simulink model "soc"  (R2025b)
settings: Solver=FixedStepDiscrete  StartTime=0.0  StopTime=10  FixedStep=0.01  RelTol=1e-3
PreLoadFcn:
  | % === Get the current model's directory ===
  | modelFullPath = get_param(bdroot, 'FileName');
  | modelDir = fileparts(modelFullPath);
  | 
  | 
  | % === Get the project root folder ===
  | projectRoot = fileparts(modelDir);
  | 
  | 
  | % === Add key folders to path ===
  | addpath(fullfile(projectRoot, 'ReferenceSubsystems'));
  | %addpath(fullfile(projectRoot, 'Docs'));
  | addpath(fullfile(projectRoot, 'design'));
  | 
  | 
  | % Load lookup table script
  | %run('Lookuptable.m');
  | 
  | 
  | 
  | 
PostLoadFcn:
  | float32 = Simulink.AliasType;
  | 
  | float32.BaseType = 'single';
  | 
  | float32.HeaderFile = 'Platform_Types.h';
  | 
  | assignin('base', 'float32', float32);
values from neighbouring files (symbols this model uses):
  Battsm_State_t : value not decoded    [soc.sldd]
  FRACTION_TO_PERCENT = 100.0    [soc.sldd]
  KeSoc_A_RestingCurrent = 4.0    [soc.sldd]
  KeSoc_frc_BotmOfDchRst = 0.0    [soc.sldd]
  KeSoc_frc_LowSocResetThd = 0.12    [soc.sldd]
  KeSoc_frc_LowSocSetThd = 0.1    [soc.sldd]
  KeSoc_frc_SocMaxLim = 1.0    [soc.sldd]
  KeSoc_frc_SocMinLim = 0.0    [soc.sldd]
  KeSoc_frc_TopOfChrgRst = 1.0    [soc.sldd]
  KeSoc_frc_UserSocMaxLim = 0.99    [soc.sldd]
  KeSoc_frc_UserSocMinLim = 0.014    [soc.sldd]
  KeSoc_nu_EpsVal = 2.2204460492503131E-16    [soc.sldd]
  KeSoc_nu_RestTauFactor = 3.0    [soc.sldd]
  KeSoc_sec_SampleTime = 0.01    [soc.sldd]
  KeSoc_sec_SocBodSetTime = 0.0    [soc.sldd]
  KeSoc_sec_SocTocSetTime = 0.0    [soc.sldd]
  KeSoc_V_BodMinCellVolt = 2.993    [soc.sldd]
  KeSoc_V_TocAvrgCellVolt = 4.5    [soc.sldd]
  KeSoc_V_TocMaxCellVolt = 4.5    [soc.sldd]
  PERCENT_TO_FRACTION = 0.01    [soc.sldd]
  SEC_TO_MILLISEC = 1000.0    [soc.sldd]
  SOC_NUM_OF_CELLS = 8.0    [soc.sldd]
  Soc_State_t : value not decoded    [soc.sldd]
libraries: simulink x25
(part 1 of 2)
settings Model: DataDictionary=soc.sldd  Creator=Niharika  LastModifiedBy=Niharika
settings OptimizationCC: BlockReduction=off  DefaultParameterBehavior=Inlined  UseDivisionForNetSlopeComputation=on  DefaultUnderspecifiedDataType=single  EnhancedBackFolding=on  PassReuseOutputArgsAs=Individual arguments  EfficientFloat2IntCast=on  LifeSpan=inf  OptimizeBlockOrder=speed  DifferentSizesBufferReuse=on  OptimizationCustomize=off  EfficientTunableParamExpr=on
settings DebuggingCC: SignalInfNanChecking=error  ReadBeforeWriteMsg=EnableAllAsError  WriteAfterWriteMsg=EnableAllAsError  WriteAfterReadMsg=EnableAllAsError  AlgebraicLoopMsg=error  ArtificialAlgebraicLoopMsg=error  SaveWithDisabledLinksMsg=error  SaveWithParameterizedLinksMsg=error  BlockPriorityViolationMsg=error  SolverPrmCheckMsg=error  SingleTaskRateTransMsg=warning  CheckMatrixSingularityMsg=error  IntegerOverflowMsg=error  ParameterOverflowMsg=none  ParameterPrecisionLossMsg=none  ParameterTunabilityLossMsg=none  UnnecessaryDatatypeConvMsg=warning  SignalLabelMismatchMsg=error  UnconnectedInputMsg=error  UnconnectedOutputMsg=error  UnconnectedLineMsg=error  SFcnCompatibilityMsg=error  UniqueDataStoreMsg=error  BusObjectLabelMismatch=error  RootOutportRequireBusObject=error  AssertControl=DisableAll  ModelReferenceIOMismatchMessage=error  ModelReferenceDataLoggingMessage=error  StateNameClashWarn=warning  StrictBusMsg=ErrorOnBusTreatedAsVector  NonBusSignalsTreatedAsBus=error  SFInvalidInputDataAccessInChartInitDiag=error  SFTransitionOutsideNaturalParentDiag=error  SFUnreachableExecutionPathDiag=error  SFUndirectedBroadcastEventsDiag=error  SFTransitionActionBeforeConditionDiag=error  SFTemporalDelaySmallerThanSampleTimeDiag=error  SFSelfTransitionDiag=error  SFExecutionAtInitializationDiag=error  IntegerSaturationMsg=error  UnderSpecifiedDimensionMsg=warning  VariantConditionMismatch=error
settings HardwareCC: ProdBitPerPointer=32.0  ProdBitPerSizeT=32.0  ProdBitPerPtrDiffT=32.0  ProdLargestAtomicInteger=Long  ProdLargestAtomicFloat=Double  ProdWordSize=32.0  ProdHWDeviceType=ARM Compatible->ARM Cortex-M
settings SFSimCC: SimGenImportedTypeDefs=on  CompileTimeRecursionLimit=0.0  EnableRuntimeRecursion=off  MATLABDynamicMemAlloc=off
settings RTWCC: SystemTargetFile=ert.tlc  GenCodeOnly=on  TemplateMakefile=ert_default_tmf  DataTypeReplacement=CDataTypesFixedWidth  GPUComputeCapability=3.5  Description=Embedded Coder
settings CodeAppCC: ForceParamTrailComments=on  IgnoreCustomStorageClasses=off  IgnoreTestpoints=on  OperatorAnnotations=on  SimulinkDataObjDesc=on  SFDataObjDesc=on  MATLABFcnDesc=on  MangleLength=4.0  CustomUserTokenString=model  InsertBlockDesc=on  ReqsInCode=on
settings ERTTargetCC: MultiInstanceErrorCode=None  ERTCustomFileTemplate=example_file_process.tlc  GlobalDataReference=InSourceFile  ERTFilePackagingFormat=Compact  PreserveExpressionOrder=on  EnableSignedLeftShifts=off  EnableSignedRightShifts=off  IndentStyle=Allman  IndentSize=4  EnableUserReplacementTypes=on  MaxIdInt64=INT64_MAX  MinIdInt64=INT64_MIN  MaxIdUint64=UINT64_MAX  MaxIdInt32=INT32_MAX  MinIdInt32=INT32_MIN  MaxIdUint32=UINT32_MAX  MaxIdInt16=INT16_MAX  MinIdInt16=INT16_MIN  MaxIdUint16=UINT16_MAX  MaxIdInt8=INT8_MAX  MinIdInt8=INT8_MIN  MaxIdUint8=UINT8_MAX  DynamicArrayContainerType=coder::array  TargetLangStandard=C99 (ISO)  GenerateFullHeader=off  IncludeMdlTerminateFcn=off  SuppressErrorStatus=on  ERTCustomFileBanners=off  SupportAbsoluteTime=off  SupportNonFinite=off  SupportComplex=off  ParenthesesLevel=Standards  CastingMode=Standards  GenerateSharedConstants=off  ERTHeaderFileRootName=$R$U$E  ERTSourceFileRootName=$R$U$E
settings ConfigComp: CovScope=ReferencedModels  DVMaxProcessTime=300.0  DVMaxTestCaseSteps=10000.0  DVTestSuiteOptimization=Auto  DVAbsoluteTolerance=1.0e-5  DVDefectChecker=off  DVDetectOutOfBounds=on  DVDesignMinMaxCheck=on  DVDetectDSMAccessViolations=on  DVDetectHISMViolationsHisl_0002=on  DVDetectHISMViolationsHisl_0003=on  DVDetectHISMViolationsHisl_0004=on  DVDetectHISMViolationsHisl_0028=on  DVDetectBlockInputRangeViolations=on  DVMaxViolationSteps=20.0  DVModelReferenceHarness=on  DVHarnessSource=Signal Editor  DVActiveTab=0.0

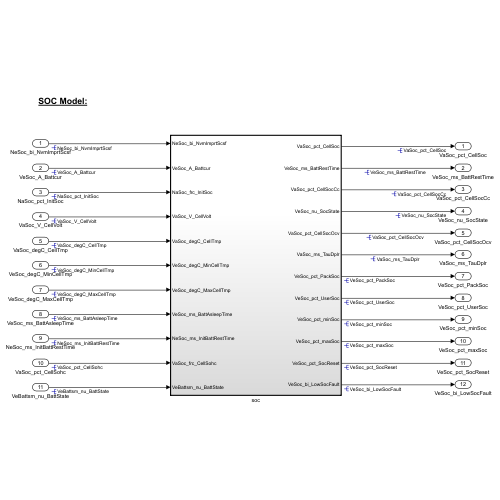
[thumbnail: Simulink's stored preview of the top-level diagram]
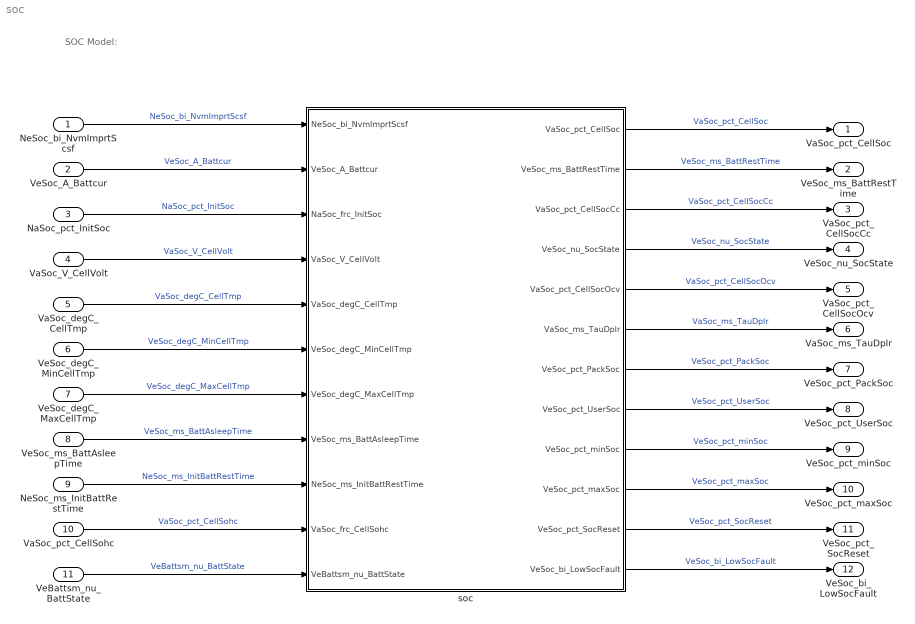
== system soc ==
  note: SOC Model:
  NeSoc_bi_NvmImprtScsf : Inport  OutMin=0  OutMax=1  OutDataTypeStr=boolean  PortDimensions=[1]  SampleTime=0.01
  VeSoc_A_Battcur : Inport  Port=2  OutMin=-6000  OutMax=6000  OutDataTypeStr=single  Unit=mA  PortDimensions=[1]  SampleTime=0.01
  NaSoc_pct_InitSoc : Inport  Port=3  OutDataTypeStr=single  PortDimensions=[1,SOC_NUM_OF_CELLS]  SampleTime=0.01
  VaSoc_V_CellVolt : Inport  Port=4  OutMin=2  OutMax=5  OutDataTypeStr=single  PortDimensions=[1,SOC_NUM_OF_CELLS]  SampleTime=0.01
  VaSoc_degC_CellTmp : Inport  Port=5  OutMin=-35  OutMax=60  OutDataTypeStr=single  Unit=degC  PortDimensions=[1,SOC_NUM_OF_CELLS]  SampleTime=0.01
  VeSoc_degC_MinCellTmp : Inport  Port=6  OutMin=-35  OutMax=60  OutDataTypeStr=single  Unit=degC  PortDimensions=[1]  SampleTime=0.01
  VeSoc_degC_MaxCellTmp : Inport  Port=7  OutMin=-35  OutMax=60  OutDataTypeStr=single  Unit=degC  PortDimensions=[1]  SampleTime=0.01
  VeSoc_ms_BattAsleepTime : Inport  Port=8  OutDataTypeStr=uint32  Unit=ms  PortDimensions=[1]  SampleTime=0.01
  NeSoc_ms_InitBattRestTime : Inport  Port=9  OutDataTypeStr=uint32  Unit=ms  PortDimensions=[1]  SampleTime=0.01
  VaSoc_pct_CellSohc : Inport  Port=10  OutMin=0.01  OutDataTypeStr=single  PortDimensions=[1,SOC_NUM_OF_CELLS]  SampleTime=0.01
  VeBattsm_nu_BattState : Inport  Port=11  OutDataTypeStr=Enum: Battsm_State_t  PortDimensions=[1]  SampleTime=0.01
  soc : Subsystem  Description=SOC Estimation Algorithm Main/Top level subsystem  TreatAsAtomicUnit=on
      settings: RTWSystemCode=Inline
  VaSoc_pct_CellSoc : Outport  OutDataTypeStr=single  PortDimensions=[1,SOC_NUM_OF_CELLS]  SampleTime=0.01
  VeSoc_ms_BattRestTime : Outport  Port=2  OutDataTypeStr=uint32  PortDimensions=[1]  SampleTime=0.01
  VaSoc_pct_CellSocCc : Outport  Port=3  OutDataTypeStr=single  PortDimensions=[1,SOC_NUM_OF_CELLS]  SampleTime=0.01
  VeSoc_nu_SocState : Outport  Port=4  OutDataTypeStr=Enum: Soc_State_t  PortDimensions=[1]  SampleTime=0.01
  VaSoc_pct_CellSocOcv : Outport  Port=5  OutDataTypeStr=single  PortDimensions=[1,SOC_NUM_OF_CELLS]  SampleTime=0.01
  VaSoc_ms_TauDplr : Outport  Port=6  OutDataTypeStr=single  PortDimensions=[1,SOC_NUM_OF_CELLS]  SampleTime=0.01
  VeSoc_pct_PackSoc : Outport  Port=7  OutDataTypeStr=single  SampleTime=0.01
  VeSoc_pct_UserSoc : Outport  Port=8  OutDataTypeStr=single  SampleTime=0.01
  VeSoc_pct_minSoc : Outport  Port=9
  VeSoc_pct_maxSoc : Outport  Port=10
  VeSoc_pct_SocReset : Outport  Port=11
  VeSoc_bi_LowSocFault : Outport  Port=12
  wires:
  soc/2(VeSoc_ms_BattRestTime) -> VeSoc_ms_BattRestTime/1  "VeSoc_ms_BattRestTime"
  soc/6(VaSoc_ms_TauDplr) -> VaSoc_ms_TauDplr/1  "VaSoc_ms_TauDplr"
  soc/3(VaSoc_pct_CellSocCc) -> VaSoc_pct_CellSocCc/1  "VaSoc_pct_CellSocCc"
  soc/5(VaSoc_pct_CellSocOcv) -> VaSoc_pct_CellSocOcv/1  "VaSoc_pct_CellSocOcv"
  soc/1(VaSoc_pct_CellSoc) -> VaSoc_pct_CellSoc/1  "VaSoc_pct_CellSoc"
  soc/4(VeSoc_nu_SocState) -> VeSoc_nu_SocState/1  "VeSoc_nu_SocState"
  soc/7(VeSoc_pct_PackSoc) -> VeSoc_pct_PackSoc/1  "VeSoc_pct_PackSoc"
  soc/8(VeSoc_pct_UserSoc) -> VeSoc_pct_UserSoc/1  "VeSoc_pct_UserSoc"
  soc/10(VeSoc_pct_maxSoc) -> VeSoc_pct_maxSoc/1  "VeSoc_pct_maxSoc"
  soc/11(VeSoc_pct_SocReset) -> VeSoc_pct_SocReset/1  "VeSoc_pct_SocReset"
  soc/12(VeSoc_bi_LowSocFault) -> VeSoc_bi_LowSocFault/1  "VeSoc_bi_LowSocFault"
  soc/9(VeSoc_pct_minSoc) -> VeSoc_pct_minSoc/1  "VeSoc_pct_minSoc"
  NeSoc_bi_NvmImprtScsf/1 -> soc/1(NeSoc_bi_NvmImprtScsf)  "NeSoc_bi_NvmImprtScsf"
  VeSoc_A_Battcur/1 -> soc/2(VeSoc_A_Battcur)  "VeSoc_A_Battcur"
  NaSoc_pct_InitSoc/1 -> soc/3(NaSoc_frc_InitSoc)  "NaSoc_pct_InitSoc"
  VaSoc_V_CellVolt/1 -> soc/4(VaSoc_V_CellVolt)  "VaSoc_V_CellVolt"
  VaSoc_degC_CellTmp/1 -> soc/5(VaSoc_degC_CellTmp)  "VaSoc_degC_CellTmp"
  VeSoc_degC_MinCellTmp/1 -> soc/6(VeSoc_degC_MinCellTmp)  "VeSoc_degC_MinCellTmp"
  VeSoc_degC_MaxCellTmp/1 -> soc/7(VeSoc_degC_MaxCellTmp)  "VeSoc_degC_MaxCellTmp"
  VeSoc_ms_BattAsleepTime/1 -> soc/8(VeSoc_ms_BattAsleepTime)  "VeSoc_ms_BattAsleepTime"
  NeSoc_ms_InitBattRestTime/1 -> soc/9(NeSoc_ms_InitBattRestTime)  "NeSoc_ms_InitBattRestTime"
  VaSoc_pct_CellSohc/1 -> soc/10(VaSoc_frc_CellSohc)  "VaSoc_pct_CellSohc"
  VeBattsm_nu_BattState/1 -> soc/11(VeBattsm_nu_BattState)  "VeBattsm_nu_BattState"

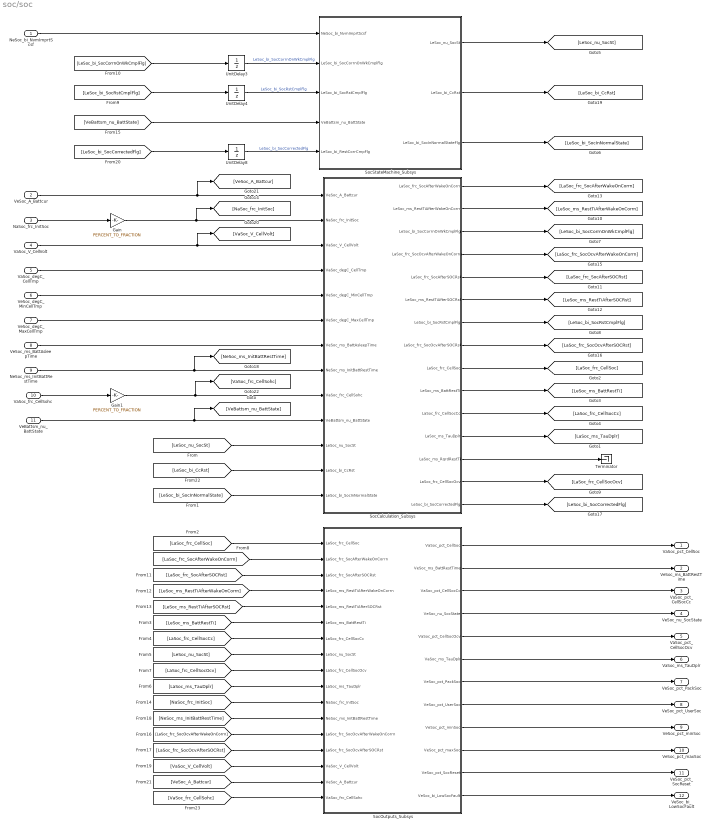
== system soc/soc ==
  NeSoc_bi_NvmImprtScsf : Inport
  VeSoc_A_Battcur : Inport  Port=2
  NaSoc_frc_InitSoc : Inport  Port=3
  VaSoc_V_CellVolt : Inport  Port=4
  VaSoc_degC_CellTmp : Inport  Port=5
  VeSoc_degC_MinCellTmp : Inport  Port=6
  VeSoc_degC_MaxCellTmp : Inport  Port=7
  VeSoc_ms_BattAsleepTime : Inport  Port=8
  NeSoc_ms_InitBattRestTime : Inport  Port=9
  VaSoc_frc_CellSohc : Inport  Port=10
  VeBattsm_nu_BattState : Inport  Port=11
  Gain : Gain  Gain=PERCENT_TO_FRACTION
  Gain1 : Gain  Gain=PERCENT_TO_FRACTION
  SocCalculation_Subsys : Subsystem  TreatAsAtomicUnit=on
  SocOutputs_Subsys : Subsystem  TreatAsAtomicUnit=on
  SocStateMachine_Subsys : Subsystem  TreatAsAtomicUnit=on
  Terminator : Terminator
  UnitDelay3 : UnitDelay  SampleTime=-1  HasFrameUpgradeWarning=on
  UnitDelay4 : UnitDelay  SampleTime=-1  HasFrameUpgradeWarning=on
  UnitDelay8 : UnitDelay  SampleTime=-1  HasFrameUpgradeWarning=on
  VaSoc_pct_CellSoc : Outport
  VeSoc_ms_BattRestTime : Outport  Port=2
  VaSoc_pct_CellSocCc : Outport  Port=3
  VeSoc_nu_SocState : Outport  Port=4
  VaSoc_pct_CellSocOcv : Outport  Port=5
  VaSoc_ms_TauDplr : Outport  Port=6
  VeSoc_pct_PackSoc : Outport  Port=7
  VeSoc_pct_UserSoc : Outport  Port=8
  VeSoc_pct_minSoc : Outport  Port=9
  VeSoc_pct_maxSoc : Outport  Port=10
  VeSoc_pct_SocReset : Outport  Port=11
  VeSoc_bi_LowSocFault : Outport  Port=12
  wires:
  NeSoc_bi_NvmImprtScsf/1 -> SocStateMachine_Subsys/1(NeSoc_bi_NvmImprtScsf)
  NaSoc_frc_InitSoc/1 -> Gain/1
  VaSoc_degC_CellTmp/1 -> SocCalculation_Subsys/4(VaSoc_degC_CellTmp)
  VeSoc_degC_MinCellTmp/1 -> SocCalculation_Subsys/5(VeSoc_degC_MinCellTmp)
  VeSoc_degC_MaxCellTmp/1 -> SocCalculation_Subsys/6(VeSoc_degC_MaxCellTmp)
  VeSoc_ms_BattAsleepTime/1 -> SocCalculation_Subsys/7(VeSoc_ms_BattAsleepTime)
  NeSoc_ms_InitBattRestTime/1 -> [NeSoc_ms_InitBattRestTime], SocCalculation_Subsys/8(NeSoc_ms_InitBattRestTime)
  VaSoc_frc_CellSohc/1 -> Gain1/1
  SocCalculation_Subsys/13(LaSoc_ms_RqrdRestTi) -> Terminator/1
  SocCalculation_Subsys/12(LaSoc_ms_TauDplr) -> [LaSoc_ms_TauDplr]
  SocCalculation_Subsys/6(LeSoc_ms_RestTiAfterSOCRst) -> [LeSoc_ms_RestTiAfterSOCRst]
  SocCalculation_Subsys/11(LaSoc_frc_CellSocCc) -> [LaSoc_frc_CellSocCc]
  SocCalculation_Subsys/10(LeSoc_ms_BattRestTi) -> [LeSoc_ms_BattRestTi]
  SocCalculation_Subsys/2(LeSoc_ms_RestTiAfterWakeOnCorrn) -> [LeSoc_ms_RestTiAfterWakeOnCorrn]
  SocCalculation_Subsys/9(LaSoc_frc_CellSoc) -> [LaSoc_frc_CellSoc]
  SocCalculation_Subsys/14(LaSoc_frc_CellSocOcv) -> [LaSoc_frc_CellSocOcv]
  SocCalculation_Subsys/7(LeSoc_bi_SocRstCmplFlg) -> [LeSoc_bi_SocRstCmplFlg]
  SocCalculation_Subsys/3(LeSoc_bi_SocCorrnOnWkCmplFlg) -> [LeSoc_bi_SocCorrnOnWkCmplFlg]
  SocStateMachine_Subsys/1(LeSoc_nu_SocSt) -> [LeSoc_nu_SocSt]
  VeSoc_A_Battcur/1 -> [VeSoc_A_Battcur], SocCalculation_Subsys/1(VeSoc_A_Battcur)
  VaSoc_V_CellVolt/1 -> [VaSoc_V_CellVolt], SocCalculation_Subsys/3(VaSoc_V_CellVolt)
  [LeSoc_ms_BattRestTi] -> SocOutputs_Subsys/6(LeSoc_ms_BattRestTi)
  SocOutputs_Subsys/5(VaSoc_pct_CellSocOcv) -> VaSoc_pct_CellSocOcv/1
  [LeSoc_ms_RestTiAfterSOCRst] -> SocOutputs_Subsys/5(LeSoc_ms_RestTiAfterSOCRst)
  [LaSoc_frc_SocAfterSOCRst] -> SocOutputs_Subsys/3(LaSoc_frc_SocAfterSOCRst)
  SocOutputs_Subsys/4(VeSoc_nu_SocState) -> VeSoc_nu_SocState/1
  [LaSoc_frc_SocAfterWakeOnCorrn] -> SocOutputs_Subsys/2(LaSoc_frc_SocAfterWakeOnCorrn)
  [LaSoc_frc_CellSocOcv] -> SocOutputs_Subsys/9(LaSoc_frc_CellSocOcv)
  [LeSoc_ms_RestTiAfterWakeOnCorrn] -> SocOutputs_Subsys/4(LeSoc_ms_RestTiAfterWakeOnCorrn)
  [LeSoc_nu_SocSt] -> SocOutputs_Subsys/8(LeSoc_nu_SocSt)
  SocOutputs_Subsys/6(VaSoc_ms_TauDplr) -> VaSoc_ms_TauDplr/1
  [LaSoc_frc_CellSoc] -> SocOutputs_Subsys/1(LaSoc_frc_CellSoc)
  SocOutputs_Subsys/3(VaSoc_pct_CellSocCc) -> VaSoc_pct_CellSocCc/1
  [LaSoc_frc_CellSocCc] -> SocOutputs_Subsys/7(LaSoc_frc_CellSocCc)
  [LaSoc_ms_TauDplr] -> SocOutputs_Subsys/10(LaSoc_ms_TauDplr)
  [LeSoc_bi_SocRstCmplFlg] -> UnitDelay4/1
  [LeSoc_bi_SocCorrnOnWkCmplFlg] -> UnitDelay3/1
  SocCalculation_Subsys/1(LaSoc_frc_SocAfterWakeOnCorrn) -> [LaSoc_frc_SocAfterWakeOnCorrn]
  SocCalculation_Subsys/5(LaSoc_frc_SocAfterSOCRst) -> [LaSoc_frc_SocAfterSOCRst]
  SocOutputs_Subsys/1(VaSoc_pct_CellSoc) -> VaSoc_pct_CellSoc/1
  SocOutputs_Subsys/2(VeSoc_ms_BattRestTime) -> VeSoc_ms_BattRestTime/1
  [VeBattsm_nu_BattState] -> SocStateMachine_Subsys/4(VeBattsm_nu_BattState)
  VeBattsm_nu_BattState/1 -> [VeBattsm_nu_BattState], SocCalculation_Subsys/10(VeBattsm_nu_BattState)
  SocCalculation_Subsys/4(LaSoc_frc_SocOcvAfterWakeOnCorrn) -> [LaSoc_frc_SocOcvAfterWakeOnCorrn]
  SocCalculation_Subsys/8(LaSoc_frc_SocOcvAfterSOCRst) -> [LaSoc_frc_SocOcvAfterSOCRst]
  [LaSoc_frc_SocOcvAfterSOCRst] -> SocOutputs_Subsys/14(LaSoc_frc_SocOcvAfterSOCRst)
  [LaSoc_frc_SocOcvAfterWakeOnCorrn] -> SocOutputs_Subsys/13(LaSoc_frc_SocOcvAfterWakeOnCorrn)
  [LeSoc_nu_SocSt] -> SocCalculation_Subsys/11(LeSoc_nu_SocSt)
  SocCalculation_Subsys/15(LeSoc_bi_SocCorrectedFlg) -> [LeSoc_bi_SocCorrectedFlg]
  [LeSoc_bi_SocCorrectedFlg] -> UnitDelay8/1
  SocStateMachine_Subsys/2(LeSoc_bi_CcRst) -> [LeSoc_bi_CcRst]
  [LeSoc_bi_CcRst] -> SocCalculation_Subsys/12(LeSoc_bi_CcRst)
  UnitDelay3/1 -> SocStateMachine_Subsys/2(LeSoc_bi_SocCorrnOnWkCmplFlg)  "LeSoc_bi_SocCorrnOnWkCmplFlg"
  UnitDelay4/1 -> SocStateMachine_Subsys/3(LeSoc_bi_SocRstCmplFlg)  "LeSoc_bi_SocRstCmplFlg"
  UnitDelay8/1 -> SocStateMachine_Subsys/5(LeSoc_bi_RestCorrCmpFlg)  "LeSoc_bi_SocCorrectedFlg"
  SocStateMachine_Subsys/3(LeSoc_bi_SocInNormalStateFlg) -> [LeSoc_bi_SocInNormalState]
  [LeSoc_bi_SocInNormalState] -> SocCalculation_Subsys/13(LeSoc_bi_SocInNormalState)
  [NaSoc_frc_InitSoc] -> SocOutputs_Subsys/11(NaSoc_frc_InitSoc)
  [NeSoc_ms_InitBattRestTime] -> SocOutputs_Subsys/12(NeSoc_ms_InitBattRestTime)
  [VaSoc_V_CellVolt] -> SocOutputs_Subsys/15(VaSoc_V_CellVolt)
  [VeSoc_A_Battcur] -> SocOutputs_Subsys/16(VeSoc_A_Battcur)
  [VaSoc_frc_CellSohc] -> SocOutputs_Subsys/17(VaSoc_frc_CellSohc)
  SocOutputs_Subsys/7(VeSoc_pct_PackSoc) -> VeSoc_pct_PackSoc/1
  SocOutputs_Subsys/8(VeSoc_pct_UserSoc) -> VeSoc_pct_UserSoc/1
  SocOutputs_Subsys/9(VeSoc_pct_minSoc) -> VeSoc_pct_minSoc/1
  SocOutputs_Subsys/10(VeSoc_pct_maxSoc) -> VeSoc_pct_maxSoc/1
  SocOutputs_Subsys/11(VeSoc_pct_SocReset) -> VeSoc_pct_SocReset/1
  SocOutputs_Subsys/12(VeSoc_bi_LowSocFault) -> VeSoc_bi_LowSocFault/1
  Gain/1 -> [NaSoc_frc_InitSoc], SocCalculation_Subsys/2(NaSoc_frc_InitSoc)
  Gain1/1 -> [VaSoc_frc_CellSohc], SocCalculation_Subsys/9(VaSoc_frc_CellSohc)

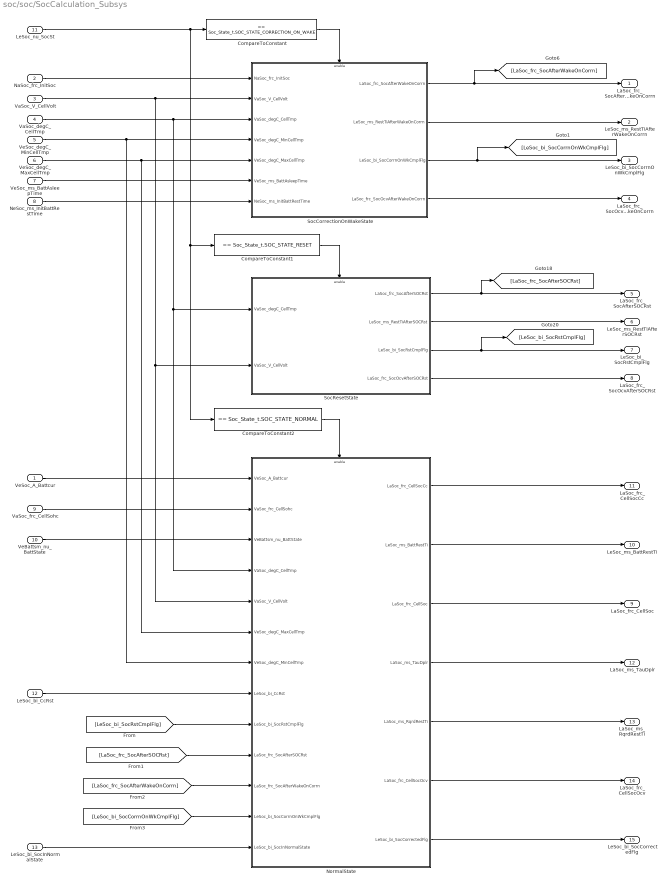
== system soc/soc/SocCalculation_Subsys ==
  VeSoc_A_Battcur : Inport
  NaSoc_frc_InitSoc : Inport  Port=2
  VaSoc_V_CellVolt : Inport  Port=3
  VaSoc_degC_CellTmp : Inport  Port=4
  VeSoc_degC_MinCellTmp : Inport  Port=5
  VeSoc_degC_MaxCellTmp : Inport  Port=6
  VeSoc_ms_BattAsleepTime : Inport  Port=7
  NeSoc_ms_InitBattRestTime : Inport  Port=8
  VaSoc_frc_CellSohc : Inport  Port=9
  VeBattsm_nu_BattState : Inport  Port=10
  LeSoc_nu_SocSt : Inport  Port=11
  LeSoc_bi_CcRst : Inport  Port=12
  LeSoc_bi_SocInNormalState : Inport  Port=13
  CompareToConstant : simulink/Logic and Bit Operations/Compare To Constant  relop===  const=Soc_State_t.SOC_STATE_CORRECTION_ON_WAKE  OutDataTypeStr=boolean
  CompareToConstant1 : simulink/Logic and Bit Operations/Compare To Constant  relop===  const=Soc_State_t.SOC_STATE_RESET  OutDataTypeStr=boolean
  CompareToConstant2 : simulink/Logic and Bit Operations/Compare To Constant  relop===  const=Soc_State_t.SOC_STATE_NORMAL  OutDataTypeStr=boolean
  NormalState : Subsystem  TreatAsAtomicUnit=on
  SocCorrectionOnWakeState : Subsystem  TreatAsAtomicUnit=on
  SocResetState : Subsystem  TreatAsAtomicUnit=on
  LaSoc_frc_SocAfterWakeOnCorrn : Outport
  LeSoc_ms_RestTiAfterWakeOnCorrn : Outport  Port=2
  LeSoc_bi_SocCorrnOnWkCmplFlg : Outport  Port=3
  LaSoc_frc_SocOcvAfterWakeOnCorrn : Outport  Port=4
  LaSoc_frc_SocAfterSOCRst : Outport  Port=5
  LeSoc_ms_RestTiAfterSOCRst : Outport  Port=6
  LeSoc_bi_SocRstCmplFlg : Outport  Port=7
  LaSoc_frc_SocOcvAfterSOCRst : Outport  Port=8
  LaSoc_frc_CellSoc : Outport  Port=9
  LeSoc_ms_BattRestTi : Outport  Port=10
  LaSoc_frc_CellSocCc : Outport  Port=11
  LaSoc_ms_TauDplr : Outport  Port=12
  LaSoc_ms_RqrdRestTi : Outport  Port=13
  LaSoc_frc_CellSocOcv : Outport  Port=14
  LeSoc_bi_SocCorrectedFlg : Outport  Port=15
  wires:
  NaSoc_frc_InitSoc/1 -> SocCorrectionOnWakeState/1(NaSoc_frc_InitSoc)
  VaSoc_V_CellVolt/1 -> SocCorrectionOnWakeState/2(VaSoc_V_CellVolt), SocResetState/2(VaSoc_V_CellVolt), NormalState/5(VaSoc_V_CellVolt)
  VaSoc_degC_CellTmp/1 -> SocCorrectionOnWakeState/3(VaSoc_degC_CellTmp), SocResetState/1(VaSoc_degC_CellTmp), NormalState/4(VaSoc_degC_CellTmp)
  VeSoc_degC_MinCellTmp/1 -> SocCorrectionOnWakeState/4(VeSoc_degC_MinCellTmp), NormalState/7(VeSoc_degC_MinCellTmp)
  VeSoc_degC_MaxCellTmp/1 -> SocCorrectionOnWakeState/5(VeSoc_degC_MaxCellTmp), NormalState/6(VeSoc_degC_MaxCellTmp)
  VeSoc_ms_BattAsleepTime/1 -> SocCorrectionOnWakeState/6(VeSoc_ms_BattAsleepTime)
  NeSoc_ms_InitBattRestTime/1 -> SocCorrectionOnWakeState/7(NeSoc_ms_InitBattRestTime)
  VeSoc_A_Battcur/1 -> NormalState/1(VeSoc_A_Battcur)
  VaSoc_frc_CellSohc/1 -> NormalState/2(VaSoc_frc_CellSohc)
  VeBattsm_nu_BattState/1 -> NormalState/3(VeBattsm_nu_BattState)
  LeSoc_nu_SocSt/1 -> CompareToConstant2/1, CompareToConstant1/1, CompareToConstant/1
  CompareToConstant/1 -> SocCorrectionOnWakeState/Enable
  CompareToConstant1/1 -> SocResetState/Enable
  CompareToConstant2/1 -> NormalState/Enable
  NormalState/6(LaSoc_frc_CellSocOcv) -> LaSoc_frc_CellSocOcv/1
  SocCorrectionOnWakeState/3(LeSoc_bi_SocCorrnOnWkCmplFlg) -> LeSoc_bi_SocCorrnOnWkCmplFlg/1, [LeSoc_bi_SocCorrnOnWkCmplFlg]
  SocResetState/3(LeSoc_bi_SocRstCmplFlg) -> LeSoc_bi_SocRstCmplFlg/1, [LeSoc_bi_SocRstCmplFlg]
  NormalState/5(LaSoc_ms_RqrdRestTi) -> LaSoc_ms_RqrdRestTi/1
  NormalState/1(LaSoc_frc_CellSocCc) -> LaSoc_frc_CellSocCc/1
  NormalState/2(LeSoc_ms_BattRestTi) -> LeSoc_ms_BattRestTi/1
  NormalState/3(LaSoc_frc_CellSoc) -> LaSoc_frc_CellSoc/1
  SocCorrectionOnWakeState/2(LeSoc_ms_RestTiAfterWakeOnCorrn) -> LeSoc_ms_RestTiAfterWakeOnCorrn/1
  SocCorrectionOnWakeState/1(LaSoc_frc_SocAfterWakeOnCorrn) -> LaSoc_frc_SocAfterWakeOnCorrn/1, [LaSoc_frc_SocAfterWakeOnCorrn]
  SocResetState/1(LaSoc_frc_SocAfterSOCRst) -> LaSoc_frc_SocAfterSOCRst/1, [LaSoc_frc_SocAfterSOCRst]
  NormalState/4(LaSoc_ms_TauDplr) -> LaSoc_ms_TauDplr/1
  SocResetState/2(LeSoc_ms_RestTiAfterSOCRst) -> LeSoc_ms_RestTiAfterSOCRst/1
  SocCorrectionOnWakeState/4(LaSoc_frc_SocOcvAfterWakeOnCorrn) -> LaSoc_frc_SocOcvAfterWakeOnCorrn/1
  SocResetState/4(LaSoc_frc_SocOcvAfterSOCRst) -> LaSoc_frc_SocOcvAfterSOCRst/1
  NormalState/7(LeSoc_bi_SocCorrectedFlg) -> LeSoc_bi_SocCorrectedFlg/1
  LeSoc_bi_CcRst/1 -> NormalState/8(LeSoc_bi_CcRst)
  [LeSoc_bi_SocRstCmplFlg] -> NormalState/9(LeSoc_bi_SocRstCmplFlg)
  [LaSoc_frc_SocAfterSOCRst] -> NormalState/10(LaSoc_frc_SocAfterSOCRst)
  [LaSoc_frc_SocAfterWakeOnCorrn] -> NormalState/11(LaSoc_frc_SocAfterWakeOnCorrn)
  [LeSoc_bi_SocCorrnOnWkCmplFlg] -> NormalState/12(LeSoc_bi_SocCorrnOnWkCmplFlg)
  LeSoc_bi_SocInNormalState/1 -> NormalState/13(LeSoc_bi_SocInNormalState)

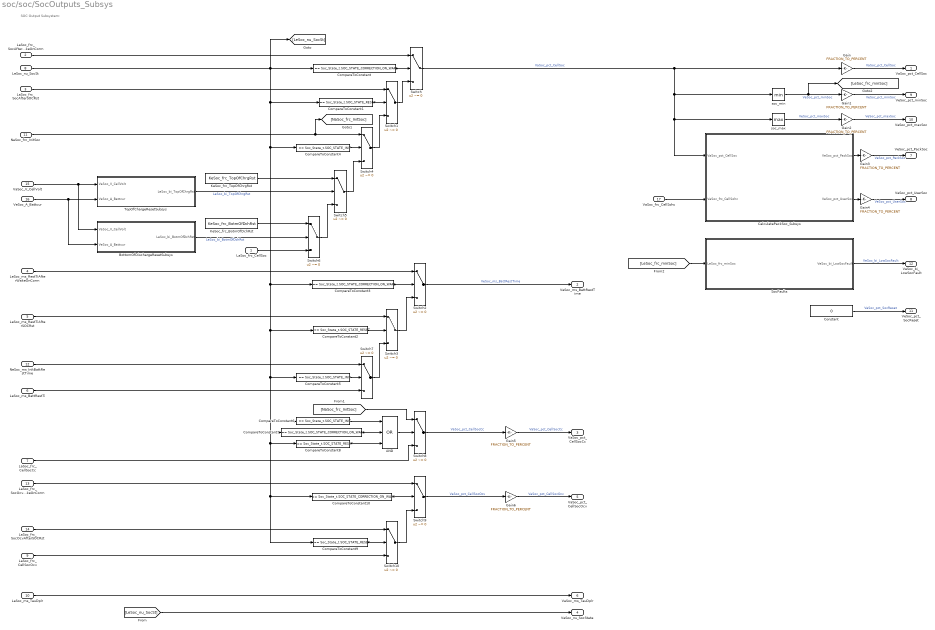
== system soc/soc/SocOutputs_Subsys ==
  note: SOC Output Subsystem:
  LaSoc_frc_CellSoc : Inport
  LaSoc_frc_SocAfterWakeOnCorrn : Inport  Port=2
  LaSoc_frc_SocAfterSOCRst : Inport  Port=3
  LeSoc_ms_RestTiAfterWakeOnCorrn : Inport  Port=4
  LeSoc_ms_RestTiAfterSOCRst : Inport  Port=5
  LeSoc_ms_BattRestTi : Inport  Port=6
  LaSoc_frc_CellSocCc : Inport  Port=7
  LeSoc_nu_SocSt : Inport  Port=8
  LaSoc_frc_CellSocOcv : Inport  Port=9
  LaSoc_ms_TauDplr : Inport  Port=10
  NaSoc_frc_InitSoc : Inport  Port=11
  NeSoc_ms_InitBattRestTime : Inport  Port=12
  LaSoc_frc_SocOcvAfterWakeOnCorrn : Inport  Port=13
  LaSoc_frc_SocOcvAfterSOCRst : Inport  Port=14
  VaSoc_V_CellVolt : Inport  Port=15
  VeSoc_A_Battcur : Inport  Port=16
  VaSoc_frc_CellSohc : Inport  Port=17
  AND : Logic  Operator=OR  Inputs=3  AllPortsSameDT=off  OutDataTypeStr=boolean
  BottomOfDischargeResetSubsys : Subsystem
  CalculatePackSoc_Subsys : Subsystem
  CompareToConstant{,3,7,10} (4 alike) : simulink/Logic and Bit Operations/Compare To Constant  relop===  const=Soc_State_t.SOC_STATE_CORRECTION_ON_WAKE  OutDataTypeStr=boolean
  CompareToConstant{1..2,8..9} (4 alike) : simulink/Logic and Bit Operations/Compare To Constant  relop===  const=Soc_State_t.SOC_STATE_RESET  OutDataTypeStr=boolean
  CompareToConstant4 : simulink/Logic and Bit Operations/Compare To Constant  relop===  const=Soc_State_t.SOC_STATE_INIT  OutDataTypeStr=boolean
  CompareToConstant5 : simulink/Logic and Bit Operations/Compare To Constant  relop===  const=Soc_State_t.SOC_STATE_INIT  OutDataTypeStr=boolean
  CompareToConstant6 : simulink/Logic and Bit Operations/Compare To Constant  relop===  const=Soc_State_t.SOC_STATE_INIT  OutDataTypeStr=boolean
  Constant : Constant  Value=0  OutDataTypeStr=single
  Gain{,1..4} (5 alike) : Gain  Gain=FRACTION_TO_PERCENT  OutDataTypeStr=single
  Gain5 : Gain  Gain=FRACTION_TO_PERCENT
  Gain6 : Gain  Gain=FRACTION_TO_PERCENT
  KeSoc_frc_BotmOfDchRst : Constant  Value=KeSoc_frc_BotmOfDchRst
  KeSoc_frc_TopOfChrgRst : Constant  Value=KeSoc_frc_TopOfChrgRst
  SocFaults : Subsystem
  Switch{,1..10} (11 alike) : Switch  Criteria=u2 ~= 0  SaturateOnIntegerOverflow=off  InputSameDT=off
  TopOfChargeResetSubsys : Subsystem
  soc_max : MinMax  Function=max
  soc_min : MinMax
  VaSoc_pct_CellSoc : Outport
  VeSoc_ms_BattRestTime : Outport  Port=2
  VaSoc_pct_CellSocCc : Outport  Port=3
  VeSoc_nu_SocState : Outport  Port=4
  VaSoc_pct_CellSocOcv : Outport  Port=5
  VaSoc_ms_TauDplr : Outport  Port=6
  VeSoc_pct_PackSoc : Outport  Port=7
  VeSoc_pct_UserSoc : Outport  Port=8
  VeSoc_pct_minSoc : Outport  Port=9
  VeSoc_pct_maxSoc : Outport  Port=10
  VeSoc_pct_SocReset : Outport  Port=11
  VeSoc_bi_LowSocFault : Outport  Port=12
  wires:
  LaSoc_ms_TauDplr/1 -> VaSoc_ms_TauDplr/1
  CompareToConstant/1 -> Switch/2
  LaSoc_frc_SocAfterWakeOnCorrn/1 -> Switch/1
  Switch1/1 -> Switch/3
  CompareToConstant1/1 -> Switch1/2
  LaSoc_frc_SocAfterSOCRst/1 -> Switch1/1
  Switch/1 -> CalculatePackSoc_Subsys/1(VaSoc_pct_CellSoc), soc_max/1, soc_min/1, Gain/1  "VaSoc_pct_CellSoc"
  CompareToConstant2/1 -> Switch3/2
  CompareToConstant3/1 -> Switch2/2
  LeSoc_ms_RestTiAfterWakeOnCorrn/1 -> Switch2/1
  LeSoc_nu_SocSt/1 -> CompareToConstant/1, CompareToConstant3/1, CompareToConstant9/1, CompareToConstant10/1, CompareToConstant8/1, CompareToConstant7/1, CompareToConstant6/1, CompareToConstant5/1, CompareToConstant2/1, CompareToConstant4/1, CompareToConstant1/1, [LeSoc_nu_SocSt]
  LeSoc_ms_RestTiAfterSOCRst/1 -> Switch3/1
  Switch4/1 -> Switch1/3
  [LeSoc_nu_SocSt] -> VeSoc_nu_SocState/1
  Switch2/1 -> VeSoc_ms_BattRestTime/1  "VeSoc_ms_BattRestTime"
  Switch3/1 -> Switch2/3
  Switch7/1 -> Switch3/3
  CompareToConstant5/1 -> Switch7/2
  NaSoc_frc_InitSoc/1 -> [NaSoc_frc_InitSoc], Switch4/1
  CompareToConstant4/1 -> Switch4/2
  LeSoc_ms_BattRestTi/1 -> Switch7/3
  NeSoc_ms_InitBattRestTime/1 -> Switch7/1
  Switch8/1 -> Gain5/1  "VaSoc_pct_CellSocCc"
  AND/1 -> Switch8/2
  CompareToConstant6/1 -> AND/1
  CompareToConstant7/1 -> AND/2
  [NaSoc_frc_InitSoc] -> Switch8/1
  LaSoc_frc_CellSocCc/1 -> Switch8/3
  CompareToConstant8/1 -> AND/3
  CompareToConstant9/1 -> Switch10/2
  LaSoc_frc_CellSocOcv/1 -> Switch10/3
  LaSoc_frc_SocOcvAfterWakeOnCorrn/1 -> Switch9/1
  Switch9/1 -> Gain6/1  "VaSoc_pct_CellSocOcv"
  CompareToConstant10/1 -> Switch9/2
  LaSoc_frc_SocOcvAfterSOCRst/1 -> Switch10/1
  Switch10/1 -> Switch9/3
  Switch5/1 -> Switch4/3
  KeSoc_frc_TopOfChrgRst/1 -> Switch5/1
  TopOfChargeResetSubsys/1(LeSoc_bi_TopOfChrgRst) -> Switch5/2  "LeSoc_bi_TopOfChrgRst"
  Switch6/1 -> Switch5/3
  KeSoc_frc_BotmOfDchRst/1 -> Switch6/1
  BottomOfDischargeResetSubsys/1(LeSoc_bi_BotmOfDchRst) -> Switch6/2  "LeSoc_bi_BotmOfDchRst"
  VaSoc_V_CellVolt/1 -> BottomOfDischargeResetSubsys/1(VaSoc_V_CellVolt), TopOfChargeResetSubsys/1(VaSoc_V_CellVolt)
  VeSoc_A_Battcur/1 -> BottomOfDischargeResetSubsys/2(VeSoc_A_Battcur), TopOfChargeResetSubsys/2(VeSoc_A_Battcur)
  LaSoc_frc_CellSoc/1 -> Switch6/3
  VaSoc_frc_CellSohc/1 -> CalculatePackSoc_Subsys/2(VaSoc_frc_CellSohc)
  CalculatePackSoc_Subsys/1(VeSoc_pct_PackSoc) -> Gain3/1
  CalculatePackSoc_Subsys/2(VeSoc_pct_UserSoc) -> Gain4/1
  soc_min/1 -> [LeSoc_frc_minSoc], Gain1/1  "VeSoc_pct_minSoc"
  soc_max/1 -> Gain2/1  "VeSoc_pct_maxSoc"
  Constant/1 -> VeSoc_pct_SocReset/1  "VeSoc_pct_SocReset"
  Gain/1 -> VaSoc_pct_CellSoc/1  "VaSoc_pct_CellSoc"
  Gain1/1 -> VeSoc_pct_minSoc/1  "VeSoc_pct_minSoc"
  Gain2/1 -> VeSoc_pct_maxSoc/1  "VeSoc_pct_maxSoc"
  Gain3/1 -> VeSoc_pct_PackSoc/1  "VeSoc_pct_PackSoc"
  Gain4/1 -> VeSoc_pct_UserSoc/1  "VeSoc_pct_UserSoc"
  Gain5/1 -> VaSoc_pct_CellSocCc/1  "VaSoc_pct_CellSocCc"
  Gain6/1 -> VaSoc_pct_CellSocOcv/1  "VaSoc_pct_CellSocOcv"
  SocFaults/1(VeSoc_bi_LowSocFault) -> VeSoc_bi_LowSocFault/1  "VeSoc_bi_LowSocFault"
  [LeSoc_frc_minSoc] -> SocFaults/1(LeSoc_frc_minSoc)

== system soc/soc/SocStateMachine_Subsys ==
  note: SOC State Machine Top Level:
  NeSoc_bi_NvmImprtScsf : Inport
  LeSoc_bi_SocCorrnOnWkCmplFlg : Inport  Port=2
  LeSoc_bi_SocRstCmplFlg : Inport  Port=3
  VeBattsm_nu_BattState : Inport  Port=4
  LeSoc_bi_RestCorrCmpFlg : Inport  Port=5
  SOC_StateMachine_Chart : Stateflow chart  TreatAsAtomicUnit=on
  LeSoc_nu_SocSt : Outport
  LeSoc_bi_CcRst : Outport  Port=2  OutDataTypeStr=boolean
  LeSoc_bi_SocInNormalStateFlg : Outport  Port=3
  wires:
  LeSoc_bi_SocRstCmplFlg/1 -> SOC_StateMachine_Chart/3(LeSoc_bi_SocRstCmplFlg)
  SOC_StateMachine_Chart/1(LeSoc_nu_SocSt) -> LeSoc_nu_SocSt/1
  LeSoc_bi_SocCorrnOnWkCmplFlg/1 -> SOC_StateMachine_Chart/2(LeSoc_bi_SocCorrnOnWkCmplFlg)
  NeSoc_bi_NvmImprtScsf/1 -> SOC_StateMachine_Chart/1(NeSoc_bi_NvmImprtScsf)
  VeBattsm_nu_BattState/1 -> SOC_StateMachine_Chart/4(VeBattsm_nu_BattState)
  LeSoc_bi_RestCorrCmpFlg/1 -> SOC_StateMachine_Chart/5(LeSoc_bi_RestCorrCmpFlg)
  SOC_StateMachine_Chart/2(LeSoc_bi_CcRst) -> LeSoc_bi_CcRst/1
  SOC_StateMachine_Chart/3(LeSoc_bi_SocInNormalStateFlg) -> LeSoc_bi_SocInNormalStateFlg/1

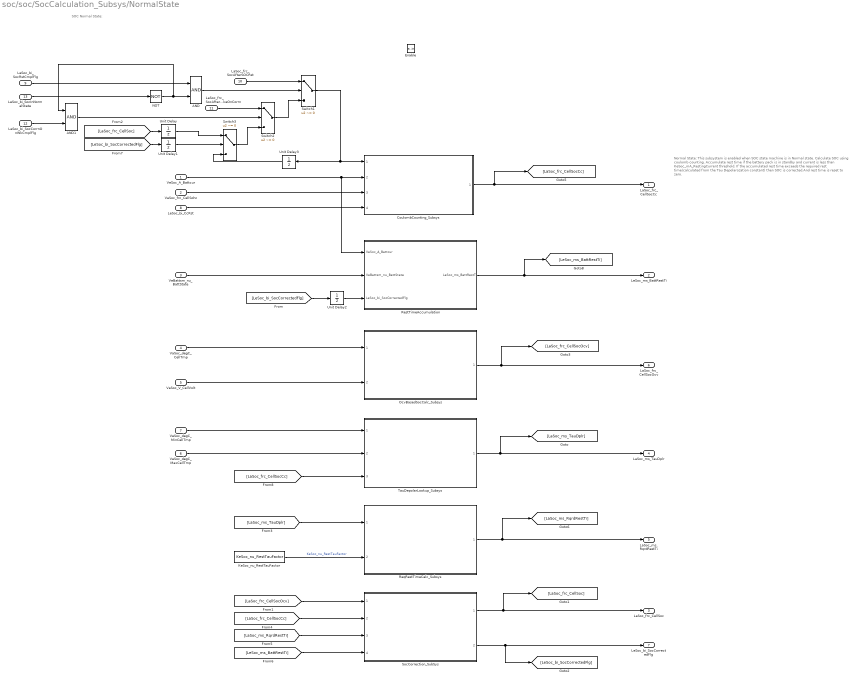
== system soc/soc/SocCalculation_Subsys/NormalState ==
  note: SOC Normal State:
  note: Normal State:
      | This subsystem is enabled when SOC state machine is in Normal state.
      | Calculate SOC using coulomb counting.
      | Accumulate rest time if the battery pack is in standby and current is less than
      | KeSoc_mA_RestingCurrent threshold.
      | If the accumulated rest time exceeds the required rest time(calculated from the Tau Depolarozation constant) then SOC is corrected.And rest time is reset to zero.
  VeSoc_A_Battcur : Inport
  VaSoc_frc_CellSohc : Inport  Port=2
  VeBattsm_nu_BattState : Inport  Port=3
  VaSoc_degC_CellTmp : Inport  Port=4
  VaSoc_V_CellVolt : Inport  Port=5
  VeSoc_degC_MaxCellTmp : Inport  Port=6
  VeSoc_degC_MinCellTmp : Inport  Port=7
  LeSoc_bi_CcRst : Inport  Port=8
  LeSoc_bi_SocRstCmplFlg : Inport  Port=9
  LaSoc_frc_SocAfterSOCRst : Inport  Port=10
  LaSoc_frc_SocAfterWakeOnCorrn : Inport  Port=11
  LeSoc_bi_SocCorrnOnWkCmplFlg : Inport  Port=12
  LeSoc_bi_SocInNormalState : Inport  Port=13
  Enable : EnablePort
  AND : Logic  AllPortsSameDT=off  OutDataTypeStr=boolean
  AND1 : Logic  AllPortsSameDT=off  OutDataTypeStr=boolean
  CoulombCounting_Subsys : Subsystem  ReferencedSubsystem=CoulombCounting_Subsys
  KeSoc_nu_RestTauFactor : Constant  Value=KeSoc_nu_RestTauFactor
  NOT : Logic  Operator=NOT  AllPortsSameDT=off  OutDataTypeStr=boolean
  OcvBasedSocCalc_Subsys : Subsystem  ReferencedSubsystem=OcvBasedSocCalc_Subsys
  ReqRestTimeCalc_Subsys : Subsystem  ReferencedSubsystem=ReqRestTimeCalc_Subsys
  RestTimeAccumulation : Subsystem
  SocCorrection_SubSys : Subsystem  ReferencedSubsystem=SocCorrection_SubSys
  Switch1 : Switch  Criteria=u2 ~= 0  SaturateOnIntegerOverflow=off  InputSameDT=off
  Switch2 : Switch  Criteria=u2 ~= 0  SaturateOnIntegerOverflow=off  InputSameDT=off
  Switch3 : Switch  Criteria=u2 ~= 0  SaturateOnIntegerOverflow=off  InputSameDT=off
  TauDepolarLookup_Subsys : Subsystem  ReferencedSubsystem=TauDepolarLookup_Subsys
  Unit Delay{,1..3} (4 alike) : UnitDelay  SampleTime=-1  HasFrameUpgradeWarning=on
  LaSoc_frc_CellSocCc : Outport
  LeSoc_ms_BattRestTi : Outport  Port=2
  LaSoc_frc_CellSoc : Outport  Port=3
  LaSoc_ms_TauDplr : Outport  Port=4
  LaSoc_ms_RqrdRestTi : Outport  Port=5
  LaSoc_frc_CellSocOcv : Outport  Port=6
  LeSoc_bi_SocCorrectedFlg : Outport  Port=7
  wires:
  VeBattsm_nu_BattState/1 -> RestTimeAccumulation/2(VeBattsm_nu_BattState)
  VaSoc_degC_CellTmp/1 -> OcvBasedSocCalc_Subsys/1
  VaSoc_V_CellVolt/1 -> OcvBasedSocCalc_Subsys/2
  VeSoc_degC_MinCellTmp/1 -> TauDepolarLookup_Subsys/1
  VeSoc_degC_MaxCellTmp/1 -> TauDepolarLookup_Subsys/2
  TauDepolarLookup_Subsys/1 -> [LaSoc_ms_TauDplr], LaSoc_ms_TauDplr/1
  SocCorrection_SubSys/1 -> [LaSoc_frc_CellSoc], LaSoc_frc_CellSoc/1
  OcvBasedSocCalc_Subsys/1 -> LaSoc_frc_CellSocOcv/1, [LaSoc_frc_CellSocOcv]
  CoulombCounting_Subsys/1 -> LaSoc_frc_CellSocCc/1, [LaSoc_frc_CellSocCc]
  ReqRestTimeCalc_Subsys/1 -> [LaSoc_ms_RqrdRestTi], LaSoc_ms_RqrdRestTi/1
  [LaSoc_frc_CellSocCc] -> TauDepolarLookup_Subsys/3
  KeSoc_nu_RestTauFactor/1 -> ReqRestTimeCalc_Subsys/2  "KeSoc_nu_RestTauFactor"
  [LaSoc_ms_RqrdRestTi] -> SocCorrection_SubSys/3
  [LeSoc_ms_BattRestTi] -> SocCorrection_SubSys/4
  [LaSoc_frc_CellSocCc] -> SocCorrection_SubSys/2
  [LaSoc_ms_TauDplr] -> ReqRestTimeCalc_Subsys/1
  [LaSoc_frc_CellSocOcv] -> SocCorrection_SubSys/1
  VeSoc_A_Battcur/1 -> RestTimeAccumulation/1(VeSoc_A_Battcur), CoulombCounting_Subsys/2
  VaSoc_frc_CellSohc/1 -> CoulombCounting_Subsys/3
  SocCorrection_SubSys/2 -> LeSoc_bi_SocCorrectedFlg/1, [LeSoc_bi_SocCorrectedFlg]
  RestTimeAccumulation/1(LeSoc_ms_BattRestTi) -> LeSoc_ms_BattRestTi/1, [LeSoc_ms_BattRestTi]
  LeSoc_bi_CcRst/1 -> CoulombCounting_Subsys/4
  Switch2/1 -> Switch1/3
  LaSoc_frc_SocAfterSOCRst/1 -> Switch1/1
  [LeSoc_bi_SocCorrectedFlg] -> Unit Delay1/1
  [LaSoc_frc_CellSoc] -> Unit Delay/1
  [LeSoc_bi_SocCorrectedFlg] -> Unit Delay2/1
  Unit Delay2/1 -> RestTimeAccumulation/3(LeSoc_bi_SocCorrectedFlg)
  LaSoc_frc_SocAfterWakeOnCorrn/1 -> Switch2/1
  Switch3/1 -> Switch2/3
  Unit Delay1/1 -> Switch3/2
  Unit Delay/1 -> Switch3/1
  Unit Delay3/1 -> Switch3/3
  Switch1/1 -> Unit Delay3/1, CoulombCounting_Subsys/1
  NOT/1 -> AND/2, AND1/1
  LeSoc_bi_SocInNormalState/1 -> NOT/1
  LeSoc_bi_SocRstCmplFlg/1 -> AND/1
  AND/1 -> Switch1/2
  AND1/1 -> Switch2/2
  LeSoc_bi_SocCorrnOnWkCmplFlg/1 -> AND1/2

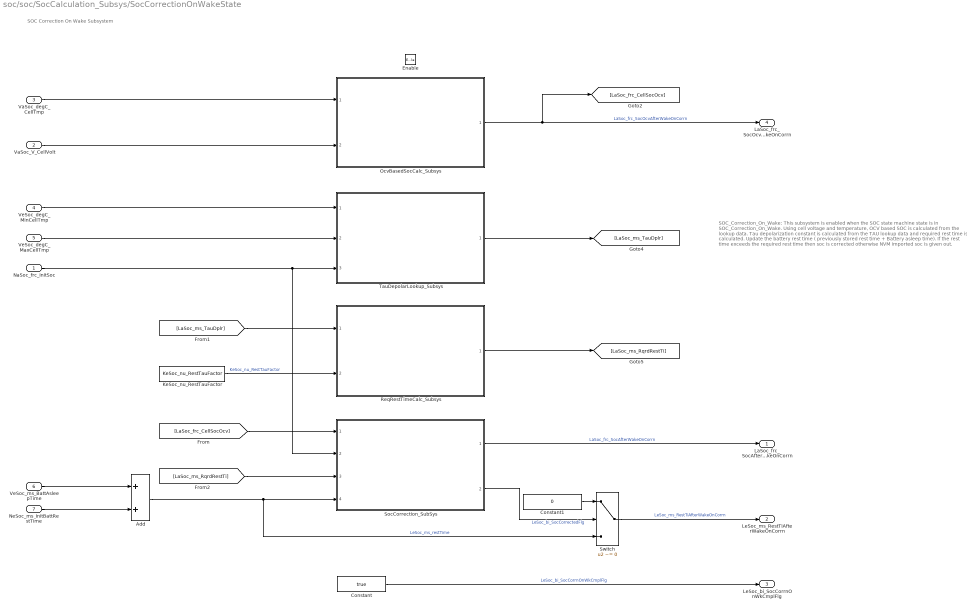
== system soc/soc/SocCalculation_Subsys/SocCorrectionOnWakeState ==
  note: SOC Correction On Wake Subsystem
  note: SOC_Correction_On_Wake:
      | This subsystem is enabled when the SOC state machine state is in SOC_Correction_On_Wake.
      | Using cell voltage and temperature, OCV based SOC is calculated from the lookup data.
      | Tau depolarization constant is calculated from the TAU lookup data and required rest time is calculated.
      | Update the battery rest time ( previously stored rest time + Battery asleep time).
      | If the rest time exceeds the required rest time then soc is corrected otherwise NVM imported soc is given out.
  NaSoc_frc_InitSoc : Inport
  VaSoc_V_CellVolt : Inport  Port=2
  VaSoc_degC_CellTmp : Inport  Port=3
  VeSoc_degC_MinCellTmp : Inport  Port=4
  VeSoc_degC_MaxCellTmp : Inport  Port=5
  VeSoc_ms_BattAsleepTime : Inport  Port=6
  NeSoc_ms_InitBattRestTime : Inport  Port=7
  Enable : EnablePort
  Add : Sum
  Constant : Constant  Value=true  OutDataTypeStr=boolean
  Constant1 : Constant  Value=0  OutDataTypeStr=uint32
  KeSoc_nu_RestTauFactor : Constant  Value=KeSoc_nu_RestTauFactor  OutDataTypeStr=single
  OcvBasedSocCalc_Subsys : Subsystem  TreatAsAtomicUnit=on  ReferencedSubsystem=OcvBasedSocCalc_Subsys
      settings: RTWSystemCode=Inline
  ReqRestTimeCalc_Subsys : Subsystem  ReferencedSubsystem=ReqRestTimeCalc_Subsys
  SocCorrection_SubSys : Subsystem  ReferencedSubsystem=SocCorrection_SubSys
  Switch : Switch  Criteria=u2 ~= 0  SaturateOnIntegerOverflow=off  InputSameDT=off
  TauDepolarLookup_Subsys : Subsystem  TreatAsAtomicUnit=on  ReferencedSubsystem=TauDepolarLookup_Subsys
      settings: RTWSystemCode=Inline
  LaSoc_frc_SocAfterWakeOnCorrn : Outport
  LeSoc_ms_RestTiAfterWakeOnCorrn : Outport  Port=2
  LeSoc_bi_SocCorrnOnWkCmplFlg : Outport  Port=3  InitialOutput=false
  LaSoc_frc_SocOcvAfterWakeOnCorrn : Outport  Port=4
  wires:
  VaSoc_degC_CellTmp/1 -> OcvBasedSocCalc_Subsys/1
  VaSoc_V_CellVolt/1 -> OcvBasedSocCalc_Subsys/2
  VeSoc_degC_MinCellTmp/1 -> TauDepolarLookup_Subsys/1
  VeSoc_degC_MaxCellTmp/1 -> TauDepolarLookup_Subsys/2
  NaSoc_frc_InitSoc/1 -> SocCorrection_SubSys/2, TauDepolarLookup_Subsys/3
  OcvBasedSocCalc_Subsys/1 -> [LaSoc_frc_CellSocOcv], LaSoc_frc_SocOcvAfterWakeOnCorrn/1  "LaSoc_frc_SocOcvAfterWakeOnCorrn"
  TauDepolarLookup_Subsys/1 -> [LaSoc_ms_TauDplr]
  ReqRestTimeCalc_Subsys/1 -> [LaSoc_ms_RqrdRestTi]
  VeSoc_ms_BattAsleepTime/1 -> Add/1
  NeSoc_ms_InitBattRestTime/1 -> Add/2
  [LaSoc_frc_CellSocOcv] -> SocCorrection_SubSys/1
  [LaSoc_ms_TauDplr] -> ReqRestTimeCalc_Subsys/1
  [LaSoc_ms_RqrdRestTi] -> SocCorrection_SubSys/3
  KeSoc_nu_RestTauFactor/1 -> ReqRestTimeCalc_Subsys/2  "KeSoc_nu_RestTauFactor"
  SocCorrection_SubSys/1 -> LaSoc_frc_SocAfterWakeOnCorrn/1  "LaSoc_frc_SocAfterWakeOnCorrn"
  Constant/1 -> LeSoc_bi_SocCorrnOnWkCmplFlg/1  "LeSoc_bi_SocCorrnOnWkCmplFlg"
  SocCorrection_SubSys/2 -> Switch/2  "LeSoc_bi_SocCorrectedFlg"
  Switch/1 -> LeSoc_ms_RestTiAfterWakeOnCorrn/1  "LeSoc_ms_RestTiAfterWakeOnCorrn"
  Constant1/1 -> Switch/1
  Add/1 -> Switch/3, SocCorrection_SubSys/4  "LeSoc_ms_restTime"

== system soc/soc/SocCalculation_Subsys/SocResetState ==
  note: SOC Reset State Subsystem:
  note: SOC Reset State:
      | This subsystem is enabled when the SOC state machine state is in SOC_Reset state.
      | SOC is updated with OCV based SOC value.
      | Reset rest time to zero.
  VaSoc_degC_CellTmp : Inport
  VaSoc_V_CellVolt : Inport  Port=2
  Enable : EnablePort
  Constant : Constant  Value=0  OutDataTypeStr=uint32
  Constant1 : Constant  Value=true  OutDataTypeStr=boolean
  OcvBasedSocCalc_Subsys : Subsystem  ReferencedSubsystem=OcvBasedSocCalc_Subsys
  LaSoc_frc_SocAfterSOCRst : Outport
  LeSoc_ms_RestTiAfterSOCRst : Outport  Port=2  InitialOutput=0
  LeSoc_bi_SocRstCmplFlg : Outport  Port=3  InitialOutput=false
  LaSoc_frc_SocOcvAfterSOCRst : Outport  Port=4
  wires:
  VaSoc_degC_CellTmp/1 -> OcvBasedSocCalc_Subsys/1
  VaSoc_V_CellVolt/1 -> OcvBasedSocCalc_Subsys/2
  OcvBasedSocCalc_Subsys/1 -> LaSoc_frc_SocOcvAfterSOCRst/1, [LaSoc_frc_CellSocOcv]
  [LaSoc_frc_CellSocOcv] -> LaSoc_frc_SocAfterSOCRst/1
  Constant/1 -> LeSoc_ms_RestTiAfterSOCRst/1  "LeSoc_ms_RestTiAfterSOCRst"
  Constant1/1 -> LeSoc_bi_SocRstCmplFlg/1  "LeSoc_bi_SocRstCmplFlg"

== system soc/soc/SocOutputs_Subsys/BottomOfDischargeResetSubsys ==
  note: Bottom of Discharge Reset Sybsystem:
  VaSoc_V_CellVolt : Inport
  VeSoc_A_Battcur : Inport  Port=2
  AND : Logic  AllPortsSameDT=off  OutDataTypeStr=boolean
  AND1 : Logic  AllPortsSameDT=off  OutDataTypeStr=boolean
  CompareToConstant : simulink/Logic and Bit Operations/Compare To Constant  relop=<  const=0  OutDataTypeStr=boolean
  CompareToConstant1 : simulink/Logic and Bit Operations/Compare To Constant  relop=<=  const=KeSoc_V_BodMinCellVolt  OutDataTypeStr=boolean
  Constant1 : Constant  Value=KeSoc_sec_SampleTime
  KeSoc_sec_SocBodSetTime : Constant  Value=KeSoc_sec_SocBodSetTime
  MinofElements : MinMax
  TimerLimit : Subsystem
  LeSoc_bi_BotmOfDchRst : Outport
  wires:
  Constant1/1 -> TimerLimit/3(dt)
  KeSoc_sec_SocBodSetTime/1 -> TimerLimit/2(TimerLimit_sec)
  AND1/1 -> LeSoc_bi_BotmOfDchRst/1
  TimerLimit/1(TimerElapsed) -> AND1/2
  VaSoc_V_CellVolt/1 -> MinofElements/1
  MinofElements/1 -> CompareToConstant1/1
  VeSoc_A_Battcur/1 -> CompareToConstant/1
  AND/1 -> AND1/1, TimerLimit/1(Enable)
  CompareToConstant/1 -> AND/2
  CompareToConstant1/1 -> AND/1

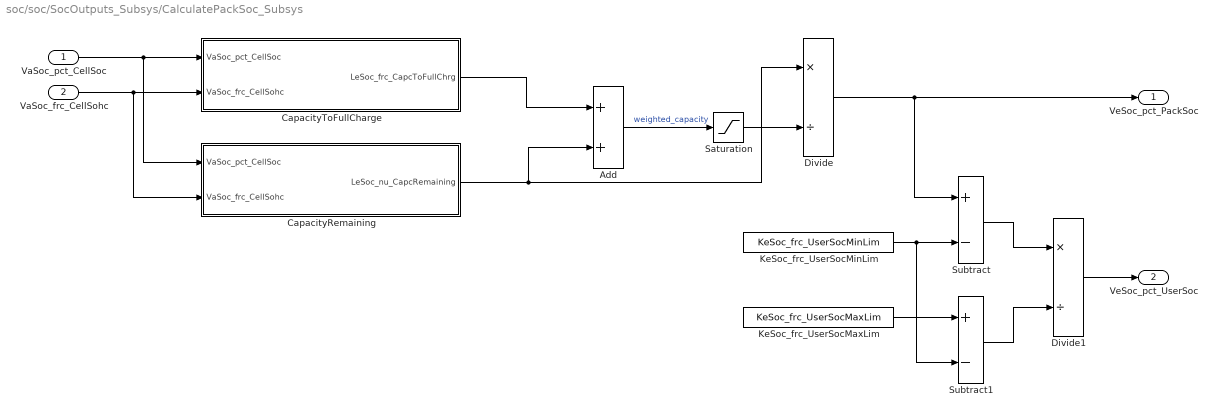
== system soc/soc/SocOutputs_Subsys/CalculatePackSoc_Subsys ==
  VaSoc_pct_CellSoc : Inport
  VaSoc_frc_CellSohc : Inport  Port=2
  Add : Sum  OutMin=0.01  OutMax=1
  CapacityRemaining : Subsystem
  CapacityToFullCharge : Subsystem
  Divide : Product  Inputs=*/
  Divide1 : Product  Inputs=*/
  KeSoc_frc_UserSocMaxLim : Constant  Value=KeSoc_frc_UserSocMaxLim
  KeSoc_frc_UserSocMinLim : Constant  Value=KeSoc_frc_UserSocMinLim
  Saturation : Saturate  UpperLimit=KeSoc_frc_SocMaxLim  LowerLimit=KeSoc_nu_EpsVal
  Subtract : Sum  Inputs=+-
  Subtract1 : Sum  Inputs=+-
  VeSoc_pct_PackSoc : Outport
  VeSoc_pct_UserSoc : Outport  Port=2
  wires:
  VaSoc_pct_CellSoc/1 -> CapacityRemaining/1(VaSoc_pct_CellSoc), CapacityToFullCharge/1(VaSoc_pct_CellSoc)
  VaSoc_frc_CellSohc/1 -> CapacityRemaining/2(VaSoc_frc_CellSohc), CapacityToFullCharge/2(VaSoc_frc_CellSohc)
  CapacityToFullCharge/1(LeSoc_frc_CapcToFullChrg) -> Add/1
  CapacityRemaining/1(LeSoc_nu_CapcRemaining) -> Divide/1, Add/2
  Divide/1 -> Subtract/1, VeSoc_pct_PackSoc/1
  Add/1 -> Saturation/1  "weighted_capacity"
  Saturation/1 -> Divide/2
  KeSoc_frc_UserSocMinLim/1 -> Subtract1/2, Subtract/2
  KeSoc_frc_UserSocMaxLim/1 -> Subtract1/1
  Subtract/1 -> Divide1/1
  Subtract1/1 -> Divide1/2
  Divide1/1 -> VeSoc_pct_UserSoc/1

== system soc/soc/SocOutputs_Subsys/SocFaults ==
  LeSoc_frc_minSoc : Inport
  AND : Logic  AllPortsSameDT=off  OutDataTypeStr=boolean
  AND1 : Logic  AllPortsSameDT=off  OutDataTypeStr=boolean
  Constant : Constant  Value=true  OutDataTypeStr=boolean
  Constant1 : Constant  Value=false  OutDataTypeStr=boolean
  KeSoc_frc_LowSocResetThd : simulink/Logic and Bit Operations/Compare To Constant  relop=>  const=KeSoc_frc_LowSocResetThd  OutDataTypeStr=boolean
  KeSoc_frc_LowSocSetThd : simulink/Logic and Bit Operations/Compare To Constant  relop=<  const=KeSoc_frc_LowSocSetThd  OutDataTypeStr=boolean
  NOT : Logic  Operator=NOT  AllPortsSameDT=off  OutDataTypeStr=boolean
  Switch : Switch  Criteria=u2 ~= 0  SaturateOnIntegerOverflow=off  InputSameDT=off
  Switch1 : Switch  Criteria=u2 ~= 0  SaturateOnIntegerOverflow=off  InputSameDT=off
  UnitDelay : UnitDelay  InitialCondition=false  SampleTime=-1  HasFrameUpgradeWarning=on
  VeSoc_bi_LowSocFault : Outport
  wires:
  UnitDelay/1 -> NOT/1, AND1/1, Switch1/3
  NOT/1 -> AND/2
  Switch/1 -> VeSoc_bi_LowSocFault/1, UnitDelay/1
  Constant1/1 -> Switch1/1
  Constant/1 -> Switch/1
  Switch1/1 -> Switch/3
  AND1/1 -> Switch1/2
  AND/1 -> Switch/2
  LeSoc_frc_minSoc/1 -> KeSoc_frc_LowSocSetThd/1, KeSoc_frc_LowSocResetThd/1
  KeSoc_frc_LowSocResetThd/1 -> AND1/2
  KeSoc_frc_LowSocSetThd/1 -> AND/1

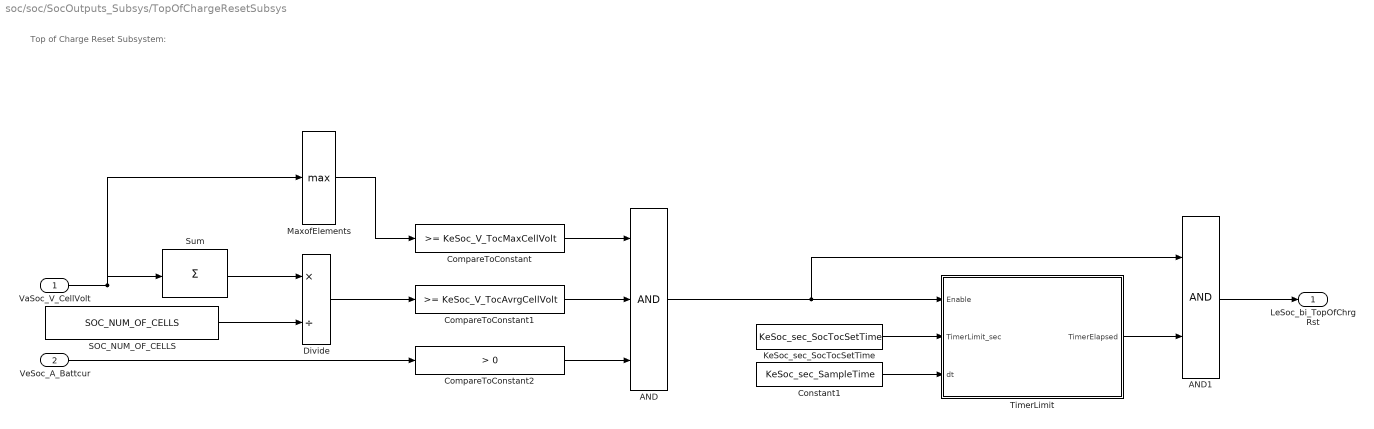
== system soc/soc/SocOutputs_Subsys/TopOfChargeResetSubsys ==
  note: Top of Charge Reset Subsystem:
  VaSoc_V_CellVolt : Inport
  VeSoc_A_Battcur : Inport  Port=2
  AND : Logic  Inputs=3  AllPortsSameDT=off  OutDataTypeStr=boolean
  AND1 : Logic  AllPortsSameDT=off  OutDataTypeStr=boolean
  CompareToConstant : simulink/Logic and Bit Operations/Compare To Constant  relop=>=  const=KeSoc_V_TocMaxCellVolt  OutDataTypeStr=boolean
  CompareToConstant1 : simulink/Logic and Bit Operations/Compare To Constant  relop=>=  const=KeSoc_V_TocAvrgCellVolt  OutDataTypeStr=boolean
  CompareToConstant2 : simulink/Logic and Bit Operations/Compare To Constant  relop=>  const=0  OutDataTypeStr=boolean
  Constant1 : Constant  Value=KeSoc_sec_SampleTime
  Divide : Product  Inputs=*/
  KeSoc_sec_SocTocSetTime : Constant  Value=KeSoc_sec_SocTocSetTime
  MaxofElements : MinMax  Function=max
  SOC_NUM_OF_CELLS : Constant  Value=SOC_NUM_OF_CELLS  OutMin=0  OutMax=1000
  Sum : Sum  Inputs=|+
  TimerLimit : Subsystem
  LeSoc_bi_TopOfChrgRst : Outport
  wires:
  VaSoc_V_CellVolt/1 -> MaxofElements/1, Sum/1
  Divide/1 -> CompareToConstant1/1
  VeSoc_A_Battcur/1 -> CompareToConstant2/1
  CompareToConstant/1 -> AND/1
  CompareToConstant1/1 -> AND/2
  CompareToConstant2/1 -> AND/3
  AND/1 -> AND1/1, TimerLimit/1(Enable)
  KeSoc_sec_SocTocSetTime/1 -> TimerLimit/2(TimerLimit_sec)
  Constant1/1 -> TimerLimit/3(dt)
  TimerLimit/1(TimerElapsed) -> AND1/2
  AND1/1 -> LeSoc_bi_TopOfChrgRst/1
  Sum/1 -> Divide/1
  MaxofElements/1 -> CompareToConstant/1
  SOC_NUM_OF_CELLS/1 -> Divide/2

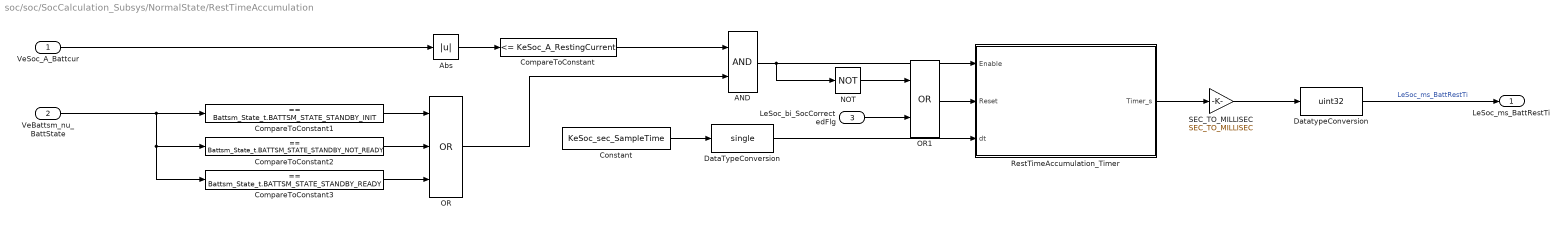
== system soc/soc/SocCalculation_Subsys/NormalState/RestTimeAccumulation ==
  VeSoc_A_Battcur : Inport
  VeBattsm_nu_BattState : Inport  Port=2
  LeSoc_bi_SocCorrectedFlg : Inport  Port=3
  AND : Logic  AllPortsSameDT=off  OutDataTypeStr=boolean
  Abs : Abs  SaturateOnIntegerOverflow=off
  CompareToConstant : simulink/Logic and Bit Operations/Compare To Constant  relop=<=  const=KeSoc_A_RestingCurrent  OutDataTypeStr=boolean
  CompareToConstant1 : simulink/Logic and Bit Operations/Compare To Constant  relop===  const=Battsm_State_t.BATTSM_STATE_STANDBY_INIT  OutDataTypeStr=boolean
  CompareToConstant2 : simulink/Logic and Bit Operations/Compare To Constant  relop===  const=Battsm_State_t.BATTSM_STATE_STANDBY_NOT_READY  OutDataTypeStr=boolean
  CompareToConstant3 : simulink/Logic and Bit Operations/Compare To Constant  relop===  const=Battsm_State_t.BATTSM_STATE_STANDBY_READY  OutDataTypeStr=boolean
  Constant : Constant  Value=KeSoc_sec_SampleTime
  DataTypeConversion : DataTypeConversion  OutDataTypeStr=single  SaturateOnIntegerOverflow=off  RndMeth=Floor
  DatatypeConversion : DataTypeConversion  OutDataTypeStr=uint32  SaturateOnIntegerOverflow=off  RndMeth=Floor
  NOT : Logic  Operator=NOT  AllPortsSameDT=off  OutDataTypeStr=boolean
  OR : Logic  Operator=OR  Inputs=3  AllPortsSameDT=off  OutDataTypeStr=boolean
  OR1 : Logic  Operator=OR  AllPortsSameDT=off  OutDataTypeStr=boolean
  RestTimeAccumulation_Timer : Subsystem
  SEC_TO_MILLISEC : Gain  Gain=SEC_TO_MILLISEC
  LeSoc_ms_BattRestTi : Outport
  wires:
  DataTypeConversion/1 -> RestTimeAccumulation_Timer/3(dt)
  Constant/1 -> DataTypeConversion/1
  VeSoc_A_Battcur/1 -> Abs/1
  AND/1 -> NOT/1, RestTimeAccumulation_Timer/1(Enable)
  Abs/1 -> CompareToConstant/1
  RestTimeAccumulation_Timer/1(Timer_s) -> SEC_TO_MILLISEC/1
  CompareToConstant/1 -> AND/1
  OR/1 -> AND/2
  CompareToConstant1/1 -> OR/1
  CompareToConstant2/1 -> OR/2
  CompareToConstant3/1 -> OR/3
  DatatypeConversion/1 -> LeSoc_ms_BattRestTi/1  "LeSoc_ms_BattRestTi"
  VeBattsm_nu_BattState/1 -> CompareToConstant3/1, CompareToConstant2/1, CompareToConstant1/1
  SEC_TO_MILLISEC/1 -> DatatypeConversion/1
  OR1/1 -> RestTimeAccumulation_Timer/2(Reset)
  NOT/1 -> OR1/1
  LeSoc_bi_SocCorrectedFlg/1 -> OR1/2
